simulink library "half_bridge_PWM_generator_with_TRGO"  (R2025b)
settings: Solver=VariableStepAuto  StartTime=0.0  StopTime=10.0  RelTol=1e-3
undefined symbols (not defined in the file): freq, tc
settings Model: Creator=dbagn  LastModifiedBy=dbagn

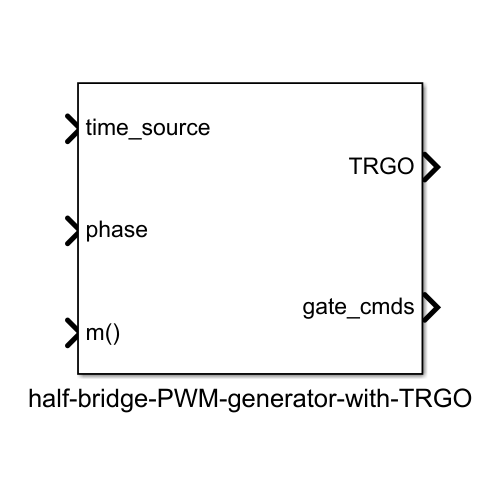
[thumbnail: Simulink's stored preview of the top-level diagram]
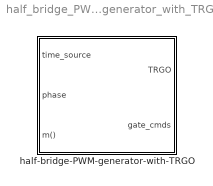
== system half_bridge_PWM_generator_with_TRGO ==
  half-bridge-PWM-generator-with-TRGO : Subsystem  mask{f=freq, m_up=0.98, m_low=0.02, dead_time=0, pos_cmd_gate=15, neg_cmd_gate=-5, polarity=1, tc=tc, double_sampling=1}
      mask prompts: f "Frequency (Hz)"; m_up "Max Input Modulation Value"; m_low "Min Input Modulation Value"; dead_time "Dead Time (s)"; pos_cmd_gate "Positive Gate Voltage (V)"; neg_cmd_gate "Negative Gate Voltage (V)"; polarity "Polarity (pu)"; tc "Sampling time"; double_sampling "Double TRGO UpDate"

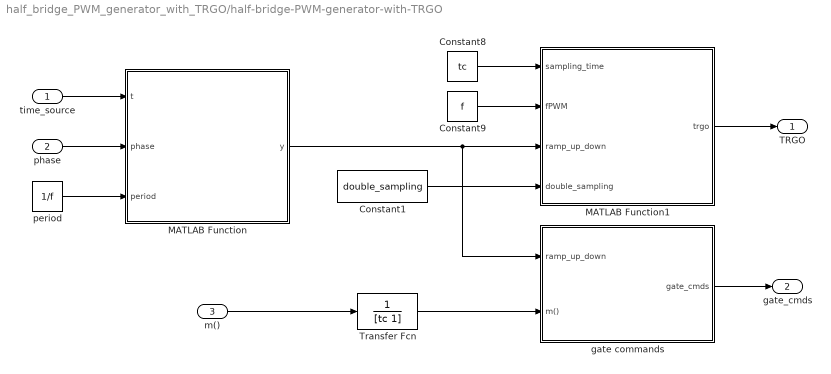
== system half_bridge_PWM_generator_with_TRGO/half-bridge-PWM-generator-with-TRGO ==
  time_source : Inport
  phase : Inport  Port=2
  m() : Inport  Port=3
  Constant1 : Constant  Value=double_sampling
  Constant8 : Constant  Value=tc
  Constant9 : Constant  Value=f
  MATLAB Function : MATLAB Function  TreatAsAtomicUnit=on  SystemSampleTime=tc
  MATLAB Function1 : MATLAB Function  TreatAsAtomicUnit=on  SystemSampleTime=tc
  Transfer Fcn : TransferFcn  Denominator=[tc 1]
  gate commands : Subsystem
  period : Constant  Value=1/f
  TRGO : Outport
  gate_cmds : Outport  Port=2
  wires:
  Constant1/1 -> MATLAB Function1/4(double_sampling)
  Transfer Fcn/1 -> gate commands/2(m())
  time_source/1 -> MATLAB Function/1(t)
  gate commands/1(gate_cmds) -> gate_cmds/1
  m()/1 -> Transfer Fcn/1
  Constant9/1 -> MATLAB Function1/2(fPWM)
  Constant8/1 -> MATLAB Function1/1(sampling_time)
  MATLAB Function1/1(trgo) -> TRGO/1
  MATLAB Function/1(y) -> MATLAB Function1/3(ramp_up_down), gate commands/1(ramp_up_down)
  phase/1 -> MATLAB Function/2(phase)
  period/1 -> MATLAB Function/3(period)

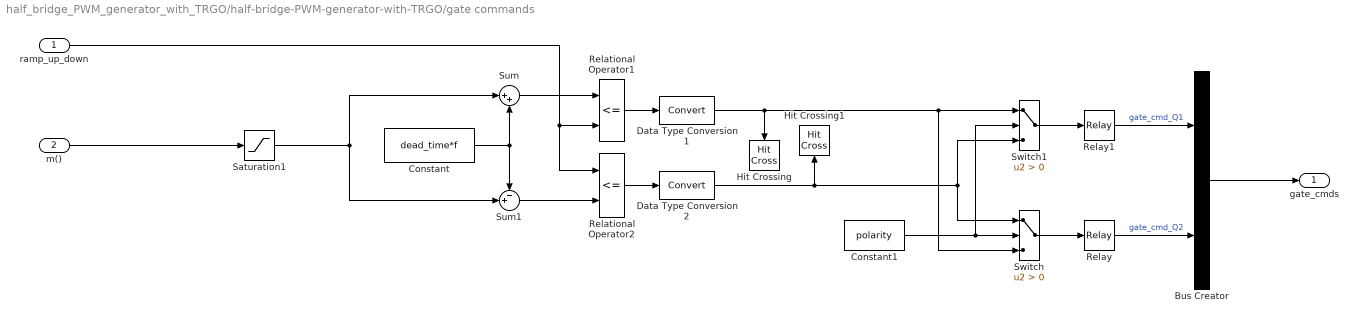
== system half_bridge_PWM_generator_with_TRGO/half-bridge-PWM-generator-with-TRGO/gate commands ==
  ramp_up_down : Inport
  m() : Inport  Port=2
  Bus Creator : BusCreator  Inputs=2
  Constant : Constant  Value=dead_time*f
  Constant1 : Constant  Value=polarity
  Data Type Conversion1 : DataTypeConversion
  Data Type Conversion2 : DataTypeConversion
  Hit Crossing : HitCross  ShowOutputPort=off
  Hit Crossing1 : HitCross  ShowOutputPort=off
  Relational Operator1 : RelationalOperator  Operator=<=  InputSameDT=off
  Relational Operator2 : RelationalOperator  Operator=<=  InputSameDT=off
  Relay : Relay  OnOutputValue=pos_cmd_gate  OffOutputValue=neg_cmd_gate
  Relay1 : Relay  OnOutputValue=pos_cmd_gate  OffOutputValue=neg_cmd_gate
  Saturation1 : Saturate  UpperLimit=m_up  LowerLimit=m_low
  Sum : Sum  Inputs=|++  SaturateOnIntegerOverflow=on
  Sum1 : Sum  Inputs=-+|  SaturateOnIntegerOverflow=on
  Switch : Switch  Criteria=u2 > Threshold  SaturateOnIntegerOverflow=off  InputSameDT=off
  Switch1 : Switch  Criteria=u2 > Threshold  SaturateOnIntegerOverflow=off  InputSameDT=off
  gate_cmds : Outport
  wires:
  m()/1 -> Saturation1/1
  Constant/1 -> Sum1/1, Sum/2
  Relay1/1 -> Bus Creator/1  "gate_cmd_Q1"
  Relay/1 -> Bus Creator/2  "gate_cmd_Q2"
  Relational Operator2/1 -> Data Type Conversion2/1
  Switch1/1 -> Relay1/1
  ramp_up_down/1 -> Relational Operator1/2, Relational Operator2/1
  Sum/1 -> Relational Operator1/1
  Switch/1 -> Relay/1
  Sum1/1 -> Relational Operator2/2
  Bus Creator/1 -> gate_cmds/1
  Relational Operator1/1 -> Data Type Conversion1/1
  Data Type Conversion2/1 -> Hit Crossing1/1, Switch1/3, Switch/1
  Saturation1/1 -> Sum/1, Sum1/2
  Data Type Conversion1/1 -> Hit Crossing/1, Switch1/1, Switch/3
  Constant1/1 -> Switch/2, Switch1/2

== matlab function half_bridge_PWM_generator_with_TRGO/half-bridge-PWM-generator-with-TRGO/MATLAB Function1 ==
  data: sampling_time input; fPWM input; ramp_up_down input; trgo output; double_sampling input
function trgo = trgo_gen(sampling_time,fPWM, ramp_up_down, double_sampling)

th = fPWM*sampling_time*2;

if double_sampling
    if (((ramp_up_down >= 0) && (ramp_up_down <= th)) || ...
            ((ramp_up_down <= 1) && (ramp_up_down >= 1-th)))
        trgo = 1;
    else
        trgo = 0;
    end
else
    if ((ramp_up_down >= 0) && (ramp_up_down <= th))
        trgo = 1;
    else
        trgo = 0;
    end
end

== matlab function half_bridge_PWM_generator_with_TRGO/half-bridge-PWM-generator-with-TRGO/MATLAB Function ==
  data: t input; y output; phase input; period input
function y = ramp_up_down(t,phase,period)
x = sin(2*pi/period*t - phase -pi/2);
y = asin(x)/pi + 1/2;
